simulink model "test"  (R2020a)
settings: Solver=VariableStepAuto  StartTime=0.0  StopTime=inf  RelTol=1e-3
values from neighbouring files (symbols this model uses):
  ts_send = 0.05    [main.m]
libraries: powerlib_meascontrol x6, instrumentlib x2, simulink x1
settings Model: Creator=bazur  LastModifiedBy=bazur

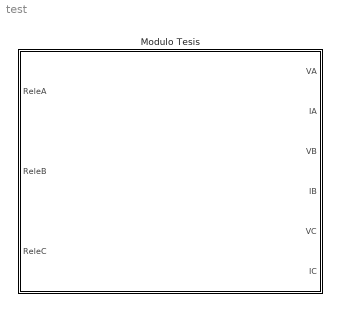
== system test ==
  Modulo Tesis : Subsystem
      mask Display: image('C:\Users\bazur\Desktop\RedNeuronal\RedNeuronalTesis\matlab\pictures\modulo.jpg'); % Use "Edit Image" on toolstrip to change.

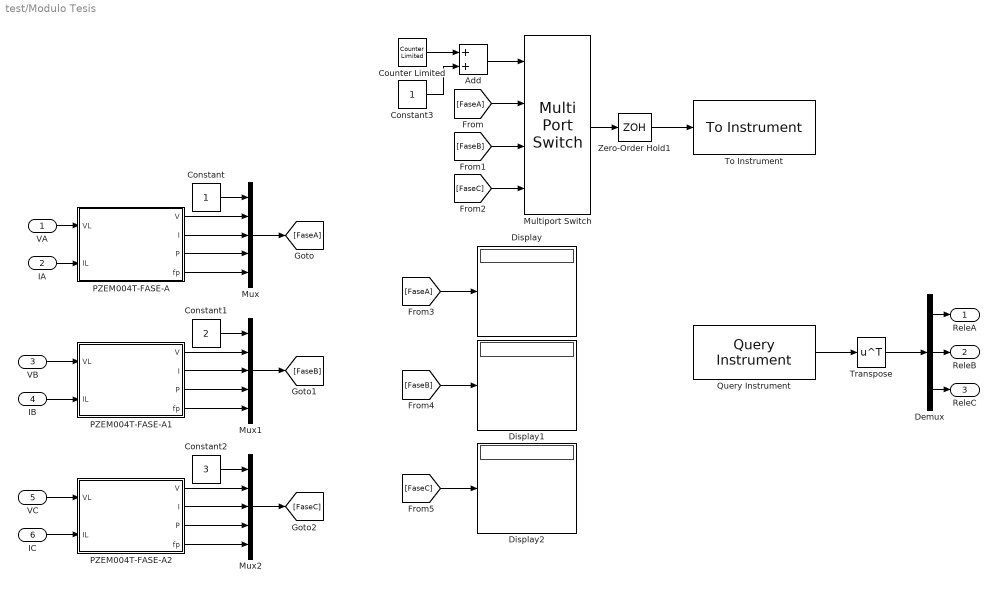
== system test/Modulo Tesis ==
  VA : Inport
  IA : Inport  Port=2
  VB : Inport  Port=3
  IB : Inport  Port=4
  VC : Inport  Port=5
  IC : Inport  Port=6
  Add : Sum
  Constant : Constant
  Constant1 : Constant  Value=2
  Constant2 : Constant  Value=3
  Constant3 : Constant
  Counter Limited : simulink/Sources/Counter Limited  uplimit=2  tsamp=ts_send
  Demux : Demux  Outputs=3
  Display : Display
  Display1 : Display
  Display2 : Display
  Multiport Switch : MultiPortSwitch
  Mux : Mux  Inputs=5
  Mux1 : Mux  Inputs=5
  Mux2 : Mux  Inputs=5
  PZEM004T-FASE-A : Subsystem
      mask Display: image('C:\Users\bazur\Desktop\RedNeuronal\RedNeuronalTesis\matlab\pictures\PZEM-004-module.jpg'); % Use "Edit Image" on toolstrip to change.
  PZEM004T-FASE-A1 : Subsystem
      mask Display: image('C:\Users\bazur\Desktop\RedNeuronal\RedNeuronalTesis\matlab\pictures\PZEM-004-module.jpg'); % Use "Edit Image" on toolstrip to change.
  PZEM004T-FASE-A2 : Subsystem
      mask Display: image('C:\Users\bazur\Desktop\RedNeuronal\RedNeuronalTesis\matlab\pictures\PZEM-004-module.jpg'); % Use "Edit Image" on toolstrip to change.
  Query Instrument : instrumentlib/Query Instrument  sampleTime=ts_read  isWorkspaceObject=off  timeout=10  inputBufferSize=1012  protocol=Serial  serialPort=COM1  baudRate=115200  gpibVendor=Keysight Technologies  boardIndex=0  primaryAddress=1  secondaryAddress=0  visaVendor=Keysight  visaSerialPort=0  chassisIndex=0  logicalAddress=0  tcpRemoteHost='127.0.0.1'  tcpRemotePort=4500  udpRemoteHost='127.0.0.1'  udpRemotePort=9090  visaTCPBoardIndex=0  visaTCPRemoteHost='127.0.0.1'  usbBoardIndex=0  usbManufID=0  usbModelCode=0  usbSerialNumber=0  initAction=None  initCommand='DATA:SOURCE CH1'  initFunction=get  queryCommand=''  responseFormat=ASCII  asciiFormatting=ASCII_read  precision=8-bit integer  byteOrder=Little endian  valuesToRead=1  removeBytes=off  afterOutputAction=Repeat query for new data  enableFrames=on  frameSize=3
      settings: SourceProductBaseCode=IC
  To Instrument : instrumentlib/To Instrument  sampleTime=ts_send  isWorkspaceObject=off  timeout=10  inputBufferSize=725000  protocol=Serial  serialPort=COM1  baudRate=115200  gpibVendor=ICS Electronics  boardIndex=0  primaryAddress=1  secondaryAddress=0  visaVendor=Keysight  visaSerialPort=0  chassisIndex=0  logicalAddress=0  tcpRemoteHost='127.0.0.1'  tcpRemotePort=4500  udpRemoteHost='127.0.0.1'  udpRemotePort=9090  visaTCPBoardIndex=0  visaTCPRemoteHost='127.0.0.1'  usbBoardIndex=0  usbManufID=0  usbModelCode=0  usbSerialNumber=0  initAction=None  initCommand='DATA:SOURCE CH1'  initFunction=get  command=''  sendFormat=ASCII  asciiFormatting=ASCII_send  precision=8-bit integer  byteOrder=Little endian
      settings: SourceProductBaseCode=IC
  Transpose : Math  Operator=transpose  SaturateOnIntegerOverflow=on
  Zero-Order Hold1 : ZeroOrderHold  SampleTime=ts_send
  ReleA : Outport
  ReleB : Outport  Port=2
  ReleC : Outport  Port=3
  wires:
  VA/1 -> PZEM004T-FASE-A/1(VL)
  IA/1 -> PZEM004T-FASE-A/2(IL)
  IB/1 -> PZEM004T-FASE-A1/2(IL)
  VB/1 -> PZEM004T-FASE-A1/1(VL)
  PZEM004T-FASE-A/1(V) -> Mux/2
  PZEM004T-FASE-A/2(I) -> Mux/3
  PZEM004T-FASE-A/3(P) -> Mux/4
  PZEM004T-FASE-A/4(fp) -> Mux/5
  Constant/1 -> Mux/1
  Mux/1 -> [FaseA]
  [FaseA] -> Multiport Switch/2
  Constant1/1 -> Mux1/1
  Mux1/1 -> [FaseB]
  PZEM004T-FASE-A1/2(I) -> Mux1/3
  PZEM004T-FASE-A1/4(fp) -> Mux1/5
  PZEM004T-FASE-A1/1(V) -> Mux1/2
  PZEM004T-FASE-A1/3(P) -> Mux1/4
  Constant2/1 -> Mux2/1
  VC/1 -> PZEM004T-FASE-A2/1(VL)
  PZEM004T-FASE-A2/3(P) -> Mux2/4
  IC/1 -> PZEM004T-FASE-A2/2(IL)
  PZEM004T-FASE-A2/4(fp) -> Mux2/5
  PZEM004T-FASE-A2/1(V) -> Mux2/2
  Mux2/1 -> [FaseC]
  PZEM004T-FASE-A2/2(I) -> Mux2/3
  [FaseB] -> Multiport Switch/3
  [FaseC] -> Multiport Switch/4
  Counter Limited/1 -> Add/1
  Add/1 -> Multiport Switch/1
  Constant3/1 -> Add/2
  Multiport Switch/1 -> Zero-Order Hold1/1
  Zero-Order Hold1/1 -> To Instrument/1
  [FaseA] -> Display/1
  [FaseB] -> Display1/1
  [FaseC] -> Display2/1
  Transpose/1 -> Demux/1
  Query Instrument/1 -> Transpose/1
  Demux/2 -> ReleB/1
  Demux/1 -> ReleA/1
  Demux/3 -> ReleC/1

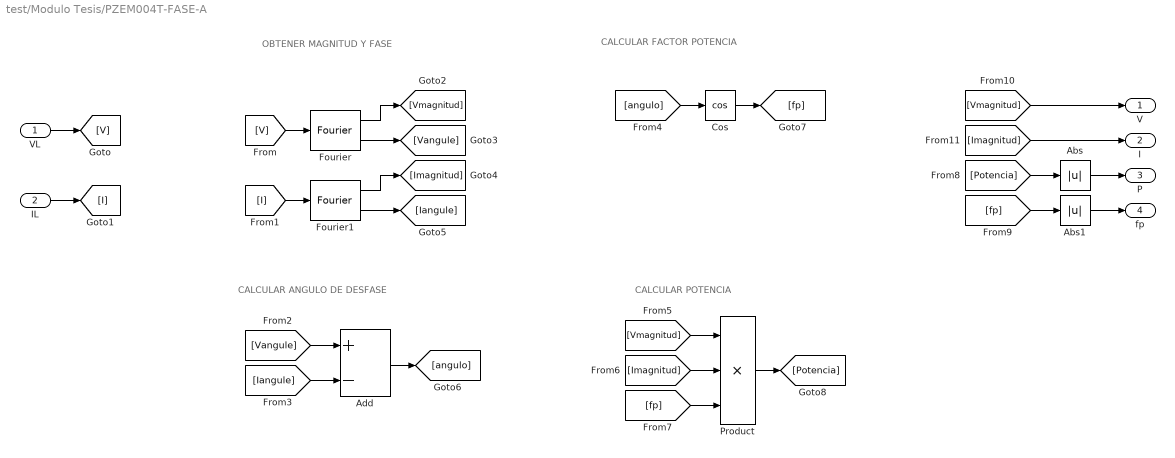
== system test/Modulo Tesis/PZEM004T-FASE-A ==
  note: OBTENER MAGNITUD Y FASE
  note: CALCULAR ANGULO DE DESFASE
  note: CALCULAR FACTOR POTENCIA
  note: CALCULAR POTENCIA
  VL : Inport
  IL : Inport  Port=2
  Abs : Abs
  Abs1 : Abs
  Add : Sum  Inputs=+-
  Cos : Trigonometry  Operator=cos
  Fourier : powerlib_meascontrol/Measurements/Fourier  Freq=60  n=1  InInit=[0, 0]  Ts=0
  Fourier1 : powerlib_meascontrol/Measurements/Fourier  Freq=60  n=1  InInit=[0, 0]  Ts=0
  Product : Product  Inputs=3
  V : Outport
  I : Outport  Port=2
  P : Outport  Port=3
  fp : Outport  Port=4
  wires:
  VL/1 -> [V]
  [V] -> Fourier/1
  IL/1 -> [I]
  [I] -> Fourier1/1
  Fourier/1 -> [Vmagnitud]
  Fourier/2 -> [Vangule]
  Fourier1/2 -> [Iangule]
  Fourier1/1 -> [Imagnitud]
  [Vangule] -> Add/1
  [Iangule] -> Add/2
  Add/1 -> [angulo]
  [angulo] -> Cos/1
  Cos/1 -> [fp]
  [Vmagnitud] -> Product/1
  [Imagnitud] -> Product/2
  [fp] -> Product/3
  Product/1 -> [Potencia]
  [Vmagnitud] -> V/1
  [Imagnitud] -> I/1
  [Potencia] -> Abs/1
  [fp] -> Abs1/1
  Abs1/1 -> fp/1
  Abs/1 -> P/1

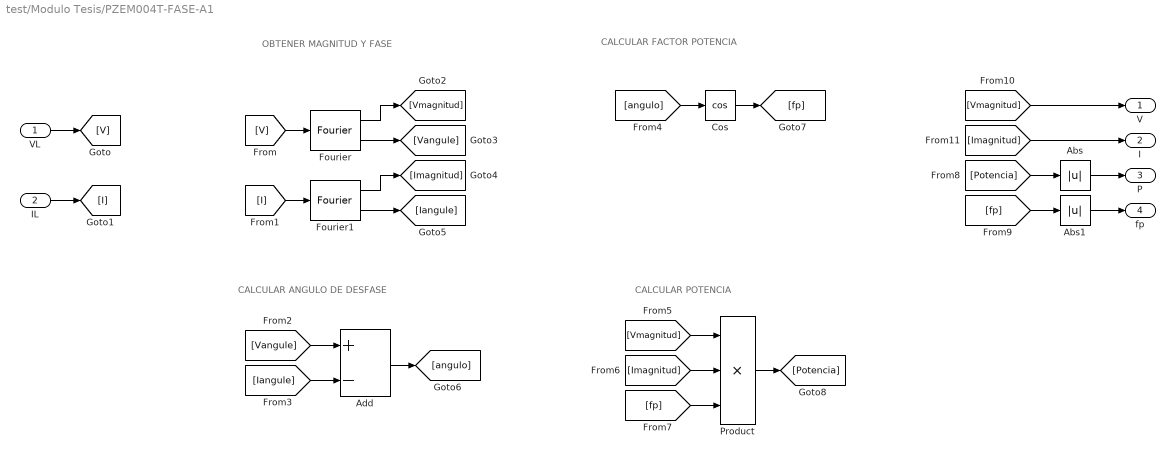
== system test/Modulo Tesis/PZEM004T-FASE-A1 ==
  note: OBTENER MAGNITUD Y FASE
  note: CALCULAR ANGULO DE DESFASE
  note: CALCULAR FACTOR POTENCIA
  note: CALCULAR POTENCIA
  VL : Inport
  IL : Inport  Port=2
  Abs : Abs
  Abs1 : Abs
  Add : Sum  Inputs=+-
  Cos : Trigonometry  Operator=cos
  Fourier : powerlib_meascontrol/Measurements/Fourier  Freq=60  n=1  InInit=[0, 0]  Ts=0
  Fourier1 : powerlib_meascontrol/Measurements/Fourier  Freq=60  n=1  InInit=[0, 0]  Ts=0
  Product : Product  Inputs=3
  V : Outport
  I : Outport  Port=2
  P : Outport  Port=3
  fp : Outport  Port=4
  wires:
  VL/1 -> [V]
  [V] -> Fourier/1
  IL/1 -> [I]
  [I] -> Fourier1/1
  Fourier/1 -> [Vmagnitud]
  Fourier/2 -> [Vangule]
  Fourier1/2 -> [Iangule]
  Fourier1/1 -> [Imagnitud]
  [Vangule] -> Add/1
  [Iangule] -> Add/2
  Add/1 -> [angulo]
  [angulo] -> Cos/1
  Cos/1 -> [fp]
  [Vmagnitud] -> Product/1
  [Imagnitud] -> Product/2
  [fp] -> Product/3
  Product/1 -> [Potencia]
  [Vmagnitud] -> V/1
  [Imagnitud] -> I/1
  [Potencia] -> Abs/1
  [fp] -> Abs1/1
  Abs1/1 -> fp/1
  Abs/1 -> P/1

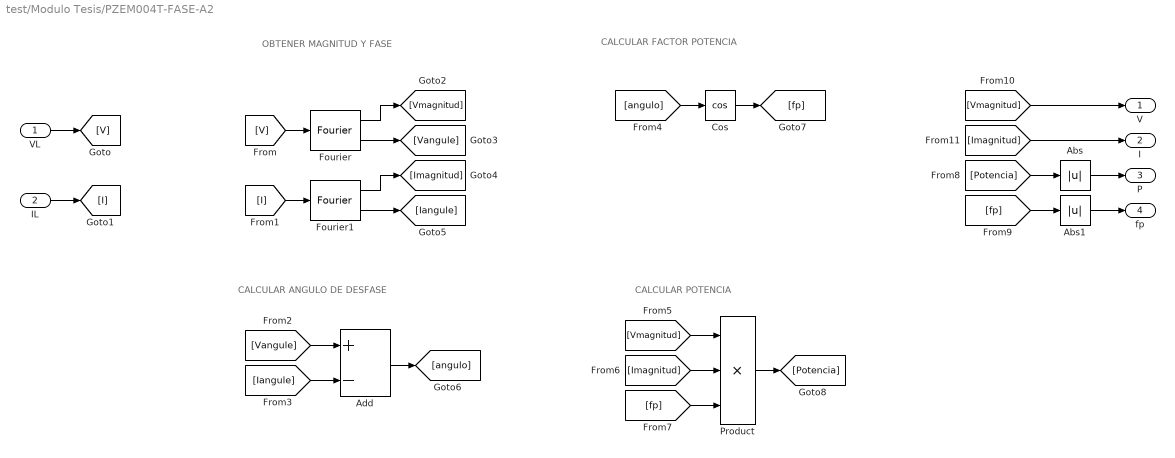
== system test/Modulo Tesis/PZEM004T-FASE-A2 ==
  note: OBTENER MAGNITUD Y FASE
  note: CALCULAR ANGULO DE DESFASE
  note: CALCULAR FACTOR POTENCIA
  note: CALCULAR POTENCIA
  VL : Inport
  IL : Inport  Port=2
  Abs : Abs
  Abs1 : Abs
  Add : Sum  Inputs=+-
  Cos : Trigonometry  Operator=cos
  Fourier : powerlib_meascontrol/Measurements/Fourier  Freq=60  n=1  InInit=[0, 0]  Ts=0
  Fourier1 : powerlib_meascontrol/Measurements/Fourier  Freq=60  n=1  InInit=[0, 0]  Ts=0
  Product : Product  Inputs=3
  V : Outport
  I : Outport  Port=2
  P : Outport  Port=3
  fp : Outport  Port=4
  wires:
  VL/1 -> [V]
  [V] -> Fourier/1
  IL/1 -> [I]
  [I] -> Fourier1/1
  Fourier/1 -> [Vmagnitud]
  Fourier/2 -> [Vangule]
  Fourier1/2 -> [Iangule]
  Fourier1/1 -> [Imagnitud]
  [Vangule] -> Add/1
  [Iangule] -> Add/2
  Add/1 -> [angulo]
  [angulo] -> Cos/1
  Cos/1 -> [fp]
  [Vmagnitud] -> Product/1
  [Imagnitud] -> Product/2
  [fp] -> Product/3
  Product/1 -> [Potencia]
  [Vmagnitud] -> V/1
  [Imagnitud] -> I/1
  [Potencia] -> Abs/1
  [fp] -> Abs1/1
  Abs1/1 -> fp/1
  Abs/1 -> P/1
